simulink model "MicroMouse2025_Template"  (R2024b)
settings: Solver=VariableStepAuto  StartTime=0.0  StopTime=10.0  RelTol=1e-3
settings Model: Creator=JesseJabezArendse  LastModifiedBy=JesseJabezArendse

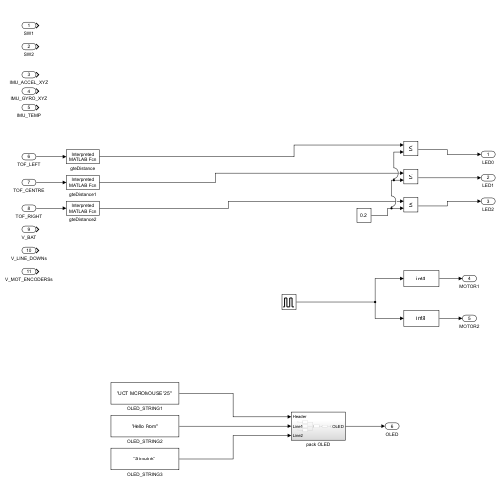
[thumbnail: Simulink's stored preview of the top-level diagram]
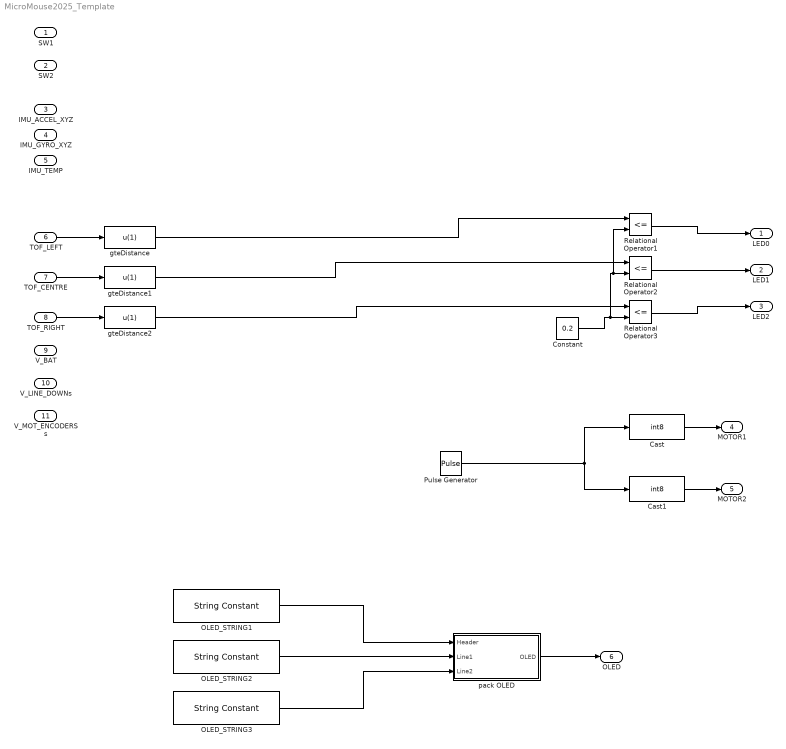
== system MicroMouse2025_Template ==
  SW1 : Inport
  SW2 : Inport  Port=2
  IMU_ACCEL_XYZ : Inport  Port=3
  IMU_GYRO_XYZ : Inport  Port=4
  IMU_TEMP : Inport  Port=5
  TOF_LEFT : Inport  Port=6
  TOF_CENTRE : Inport  Port=7
  TOF_RIGHT : Inport  Port=8
  V_BAT : Inport  Port=9
  V_LINE_DOWNs : Inport  Port=10
  V_MOT_ENCODERSs : Inport  Port=11
  Cast : DataTypeConversion  OutDataTypeStr=int8  SaturateOnIntegerOverflow=off  RndMeth=Floor
  Cast1 : DataTypeConversion  OutDataTypeStr=int8  SaturateOnIntegerOverflow=off  RndMeth=Floor
  Constant : Constant  Value=0.2
  OLED_STRING1 : StringConstant  String="\"UCT MICROMOUSE '25\""
  OLED_STRING2 : StringConstant  String="\"Hello From\""
  OLED_STRING3 : StringConstant  String="\"Simulink\""
  Pulse Generator : DiscretePulseGenerator  PulseType=Time based  Amplitude=70  Period=0.5  PulseWidth=50
  Relational Operator1 : RelationalOperator  Operator=<=  OutDataTypeStr=boolean  RndMeth=Simplest  InputSameDT=off
  Relational Operator2 : RelationalOperator  Operator=<=  OutDataTypeStr=boolean  RndMeth=Simplest  InputSameDT=off
  Relational Operator3 : RelationalOperator  Operator=<=  OutDataTypeStr=boolean  RndMeth=Simplest  InputSameDT=off
  gteDistance : MATLABFcn  MATLABFcn=u(1)  OutputDimensions=1
  gteDistance1 : MATLABFcn  MATLABFcn=u(1)  OutputDimensions=1
  gteDistance2 : MATLABFcn  MATLABFcn=u(1)  OutputDimensions=1
  pack OLED : Subsystem
  LED0 : Outport
  LED1 : Outport  Port=2
  LED2 : Outport  Port=3
  MOTOR1 : Outport  Port=4
  MOTOR2 : Outport  Port=5
  OLED : Outport  Port=6
  wires:
  OLED_STRING1/1 -> pack OLED/1(Header)
  Pulse Generator/1 -> Cast1/1, Cast/1
  Relational Operator2/1 -> LED1/1
  Cast/1 -> MOTOR1/1
  pack OLED/1(OLED) -> OLED/1
  gteDistance1/1 -> Relational Operator2/1
  TOF_LEFT/1 -> gteDistance/1
  Relational Operator1/1 -> LED0/1
  OLED_STRING3/1 -> pack OLED/3(Line2)
  Relational Operator3/1 -> LED2/1
  gteDistance/1 -> Relational Operator1/1
  gteDistance2/1 -> Relational Operator3/1
  OLED_STRING2/1 -> pack OLED/2(Line1)
  TOF_RIGHT/1 -> gteDistance2/1
  Cast1/1 -> MOTOR2/1
  TOF_CENTRE/1 -> gteDistance1/1
  Constant/1 -> Relational Operator1/2, Relational Operator2/2, Relational Operator3/2

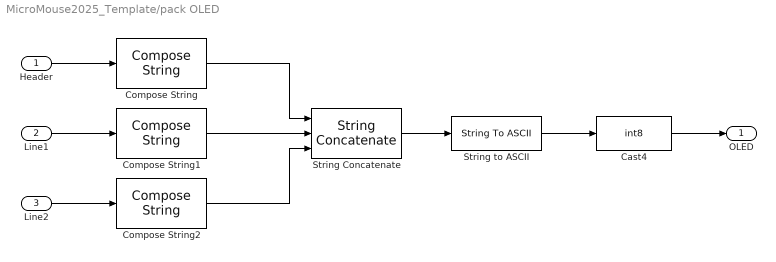
== system MicroMouse2025_Template/pack OLED ==
  Header : Inport
  Line1 : Inport  Port=2
  Line2 : Inport  Port=3
  Cast4 : DataTypeConversion  OutDataTypeStr=int8  SaturateOnIntegerOverflow=off  RndMeth=Floor
  Compose String : ComposeString  Format="\"%-18s\""
  Compose String1 : ComposeString  Format="\"%-11s\""
  Compose String2 : ComposeString  Format="\"%-11s\""
  String Concatenate : StringConcatenate  Inputs=3
  String to ASCII : StringToASCII  OutputVectorSize=18+11+11
  OLED : Outport
  wires:
  String to ASCII/1 -> Cast4/1
  Compose String/1 -> String Concatenate/1
  Line1/1 -> Compose String1/1
  String Concatenate/1 -> String to ASCII/1
  Line2/1 -> Compose String2/1
  Compose String2/1 -> String Concatenate/3
  Compose String1/1 -> String Concatenate/2
  Header/1 -> Compose String/1
  Cast4/1 -> OLED/1
